simulink model "loopshape"  (Simulink 8.0)
settings: Solver=ode45  StartTime=0.0  StopTime=10.0  RelTol=1e-3
values from neighbouring files (symbols this model uses):
  Cs = 0.3    [test2.m]
settings Model: Creator=felipe  LastModifiedBy=LabControl
settings OptimizationCC: ExpressionDepthLimit=128
settings DebuggingCC: UnderspecifiedInitializationDetection=Simplified  MergeDetectMultiDrivingBlocksExec=error  FrameProcessingCompatibilityMsg=error  StateNameClashWarn=none
settings HardwareCC: TargetIntDivRoundTo=Zero  TargetEndianess=LittleEndian  TargetHWDeviceType=MATLAB Host  ProdEqTarget=off
settings RTWCC: SystemTargetFile=rtwsfcn.tlc  TemplateMakefile=rtwsfcn_default_tmf  Description=S-Function Target  ProcessScript=rtwsfcn_make_rtw_hook  TargetLang=C++
settings CodeAppCC: CustomSymbolStrType=$N$R$M_T  InternalIdentifier=Shortened
settings STFCustomTargetCC: ModelReferenceCompliant=off  CompOptLevelCompliant=on  SystemTargetFile=rtwsfcn.tlc
settings CustomProperty: Value=on

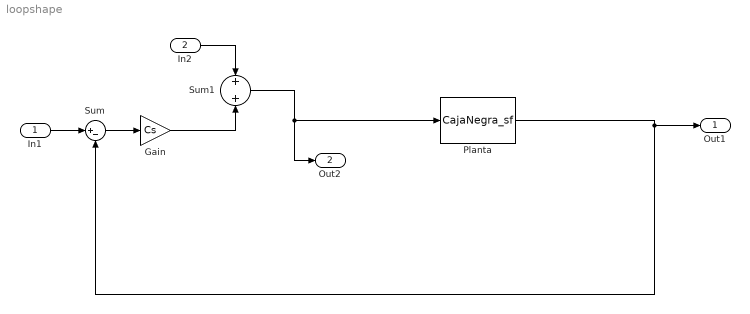
== system loopshape ==
  In1 : Inport
  In2 : Inport  Port=2
  Gain : Gain  Gain=Cs
  Planta : S-Function  FunctionName=CajaNegra_sf  EnableBusSupport=off
  Sum : Sum  Inputs=|+-
  Sum1 : Sum
  Out1 : Outport
  Out2 : Outport  Port=2
  wires:
  Sum/1 -> Gain/1
  In1/1 -> Sum/1
  In2/1 -> Sum1/1
  Gain/1 -> Sum1/2
  Sum1/1 -> Out2/1, Planta/1
  Planta/1 -> Out1/1, Sum/2
